simulink model "AS_ExhalationCircuit_VerifierModel"  (R2022b)
settings: Solver=VariableStepAuto  StartTime=0.0  StopTime=10.0  RelTol=1e-3
undefined symbols (not defined in the file): PIDiameter
libraries: fl_lib x2, nesl_utility x2, simulink x1
settings Model: DataDictionary=AS_DataDictionary.sldd  Creator=CSN-Simulation  LastModifiedBy=MATLAB
settings DebuggingCC: UnconnectedInputMsg=warning  UnconnectedOutputMsg=warning  UnconnectedLineMsg=warning
settings ModelReferenceCC: EnableRefExpFcnMdlSchedulingChecks=on
settings RTWCC: DLArmComputeVersion=19.05

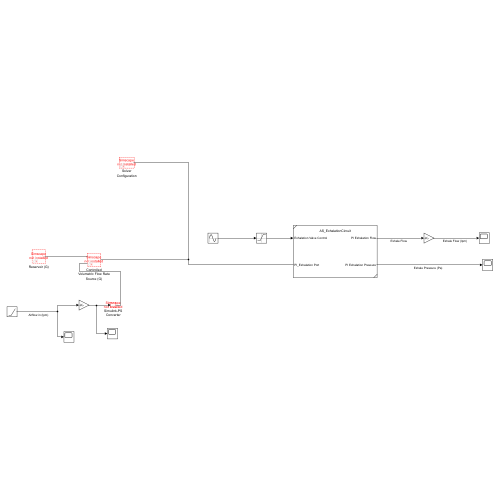
[thumbnail: Simulink's stored preview of the top-level diagram]
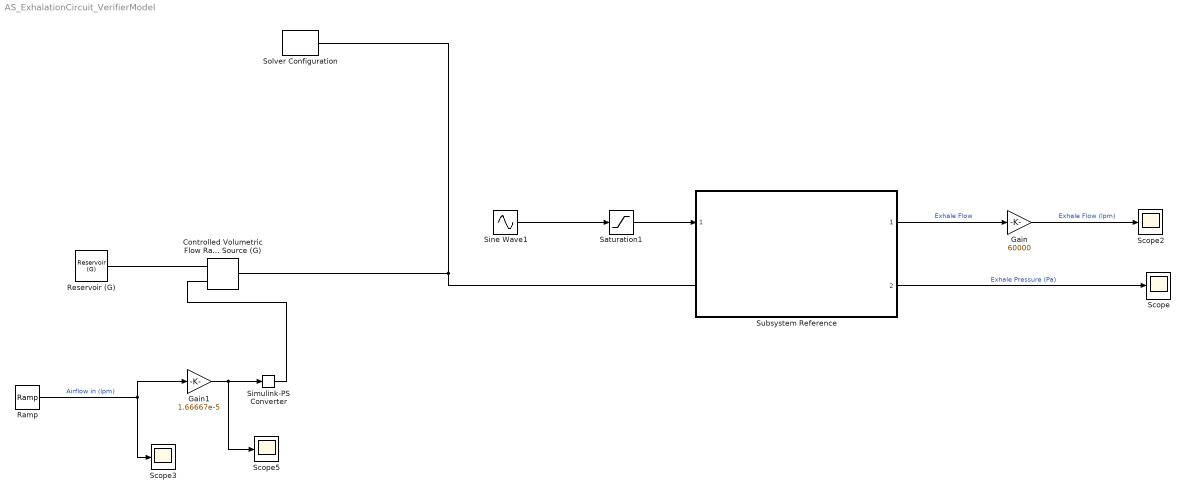
== system AS_ExhalationCircuit_VerifierModel ==
  Controlled Volumetric Flow Rate Source (G) : fl_lib/Gas/Sources/Controlled Volumetric Flow Rate Source (G)  power_spec=foundation.enum.power_spec.isentropic  area_A=pi*(PIDiameter/2)^2 mm^2  area_B=pi*(PIDiameter/2)^2 mm^2
      settings: InternalSimscapePortConfiguration="{\"Bottom\":[],\"Left\":[{\"id\":\"A\",\"label\":\"A\",\"type\":\"foundation.gas.gas\"},{\"id\":\"V\",\"label\":\"V\",\"type\":\"input\"}],\"Right\":[{\"id\":\"B\",\"label\":\"B\",\"type\":\"foundation.gas.gas\"}],\"Top\":[]}"
  Gain : Gain  Gain=60000
  Gain1 : Gain  Gain=1.66667e-5
  Ramp : simulink/Sources/Ramp  slope=1  start=0  InitialOutput=1
  Reservoir (G) : fl_lib/Gas/Elements/Reservoir (G)  pressure_spec=foundation.enum.pressure_spec.atmospheric  reservoir_pressure=0.101325 MPa  reservoir_temperature=T_room degC  area_A=pi*(PIDiameter/2)^2 mm^2
  Saturation1 : Saturate  UpperLimit=1  LowerLimit=0.0000001
  Scope{,2..3,5} (4 alike) : Scope
  Simulink-PS Converter : nesl_utility/Simulink-PS Converter  PhysicalDomain=network_engine_domain  SubClassName=ps_input  LeftPortType=input  RightPortType=output  PseudoPeriodic=off  Frequencies=[]  NoiseDistribution=none  NoiseParameters=[]  Unit=m^3/s  AffineConversion=off  FilteringAndDerivatives=provide  SimscapeFilterOrder=1  InputFilterTimeConstant=0.001  UdotUserProvided=0
  Sine Wave1 : Sin  Amplitude=0.000464  Frequency=0.5  SampleTime=0
  Solver Configuration : nesl_utility/Solver Configuration  PhysicalDomain=network_engine_domain  SubClassName=solver  LeftPortType=input  RightPortType=generic  Tones=[]  Harmonics=[]  SimulateNoise=off  Profile=off  UseLocalSampling=off  EnableSwitchedLinearOptims=on  FrequencyDomain=off  UseCCode=off  RelTol=0.001  AbsTol=1e-06  MinStep=1e-09  ToWorkspace=off  RevertToSquareIcSolve=off  NumHomotopyIterations=100  PhasorMode=off  PhasorModeNumHarmonics=1  DoDC=off  ResidualTolerance=1e-09  UseLocalSolver=off  LocalSolverChoice=NE_BACKWARD_EULER_ADVANCER  LocalSolverSampleTime=0.001  DoFixedCost=off  MaxNonlinIter=3  MaxModeIter=2  ComputeImpulses=off  ImpulseIterations=2  LinearAlgebra=auto  EquationFormulation=NE_TIME_EF  DelaysMemoryBudget=1024  AutomaticFiltering=on  FilteringTimeConstant=0.001  PartitionStorageMethod=AS_NEEDED  PartitionMemoryBudget=1024  PartitionMethod=ROBUST
  Subsystem Reference : Subsystem  ReferencedSubsystem=AS_ExhalationCircuit
  wires:
  Subsystem Reference/2 -> Scope/1  "Exhale Pressure (Pa)"
  Subsystem Reference/1 -> Gain/1  "Exhale Flow"
  Gain/1 -> Scope2/1  "Exhale Flow (lpm)"
  Sine Wave1/1 -> Saturation1/1
  Saturation1/1 -> Subsystem Reference/1
  Gain1/1 -> Scope5/1, Simulink-PS Converter/1
  Ramp/1 -> Gain1/1, Scope3/1  "Airflow in (lpm)"
  connections:
  Solver Configuration/RConn1 -- Controlled Volumetric Flow Rate Source (G)/RConn1 -- Subsystem Reference/LConn1
  Controlled Volumetric Flow Rate Source (G)/LConn1 -- Reservoir (G)/LConn1
  Controlled Volumetric Flow Rate Source (G)/LConn2 -- Simulink-PS Converter/RConn1
